simulink model "lab7_t22"  (R2021a)
settings: Solver=VariableStepAuto  StartTime=0.0  StopTime=10.0  RelTol=1e-3
settings Model: Creator=reemb  LastModifiedBy=reemb

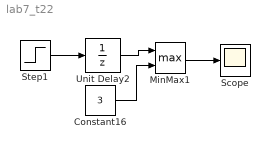
== system lab7_t22 ==
  Constant16 : Constant  Value=3
  MinMax1 : MinMax  Function=max  Inputs=2
  Scope : Scope
  Step1 : Step  Time=2  After=10  SampleTime=0
  Unit Delay2 : UnitDelay  HasFrameUpgradeWarning=on
  wires:
  Step1/1 -> Unit Delay2/1
  Constant16/1 -> MinMax1/2
  Unit Delay2/1 -> MinMax1/1
  MinMax1/1 -> Scope/1
